simulink model "code"  (R2021b)
settings: Solver=FixedStepAuto  StartTime=0.0  StopTime=inf  RelTol=1e-3  EnableMultiTasking=on
libraries: vexarmcortexlib x5, vexcommonlib x2
settings Model: PacingRate=0.110000  Creator=mukul  LastModifiedBy=mukul
settings DataIOCC: LimitDataPoints=on  SignalLoggingSaveFormat=ModelDataLogs  ReturnWorkspaceOutputs=off
settings OptimizationCC: ExpressionDepthLimit=2147483647  LifeSpan=Inf  MaxStackSize=64  EfficientTunableParamExpr=on
settings DebuggingCC: UnderspecifiedInitializationDetection=Classic  MergeDetectMultiDrivingBlocksExec=none  InheritedTsInSrcMsg=none  FcnCallInpInsideContextMsg=warning  UnconnectedInputMsg=none  UnconnectedOutputMsg=none  StateNameClashWarn=warning  SFUnexpectedBacktrackingDiag=warning  SFNoUnconditionalDefaultTransitionDiag=warning  SFExecutionAtInitializationDiag=none  SFMachineParentedDataDiag=warning  ArithmeticOperatorsInVariantConditions=warning
settings HardwareCC: ProdBitPerPointer=32  ProdBitPerSizeT=32  ProdBitPerPtrDiffT=32  ProdLargestAtomicInteger=Long  ProdLargestAtomicFloat=Double  ProdIntDivRoundTo=Undefined  ProdWordSize=32  ProdHWDeviceType=ARM Compatible->ARM Cortex
settings ModelReferenceCC: PropagateSignalLabelsOutOfModel=off
settings SFSimCC: MATLABDynamicMemAlloc=off  CustomCodeUndefinedFunction=UseInterfaceOnly
settings RTWCC: Description=Embedded Coder  SystemTargetFile=ert.tlc  HardwareBoard=ARM Cortex-based VEX Microcontroller  TemplateMakefile=ert_default_tmf  Toolchain=GNU Tools for VEX ARM Cortex
settings CodeAppCC: IgnoreCustomStorageClasses=off  CustomSymbolStrType=$N$R$M  StateflowObjectComments=on  InternalIdentifier=Classic
settings ERTTargetCC: CodeReplacementLibrary=GCC ARM Cortex-M3  MultiwordLength=2048  ConvertIfToSwitch=off  SuppressUnreachableDefaultCases=off

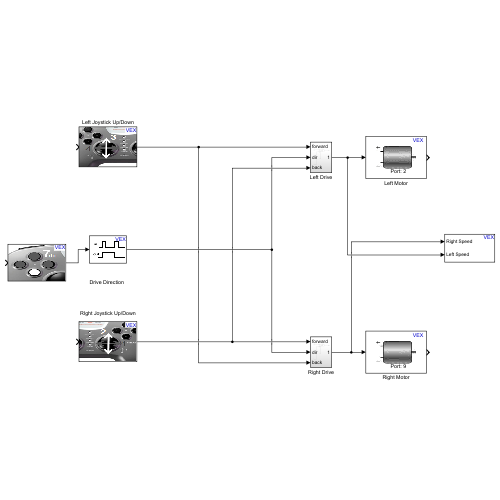
[thumbnail: Simulink's stored preview of the top-level diagram]
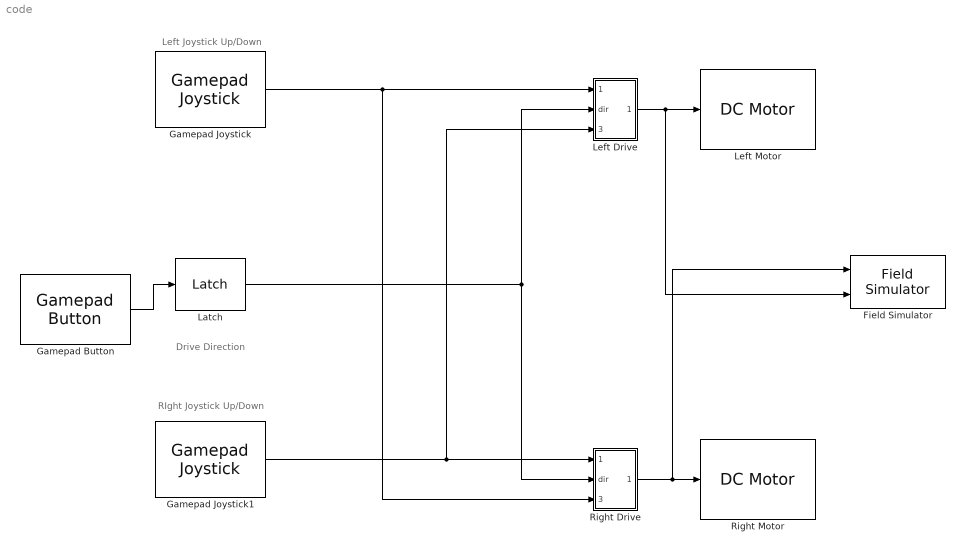
== system code ==
  note: RIght Joystick Up/Down
  note: Left Joystick Up/Down
  note: Drive Direction
  Field Simulator : vexcommonlib/Field Simulator  radius=2.5  space=10  range=200  BlockPlatform=vexarmcortex
      settings: SourceProductBaseCode=EC_VEX_MICRO,VEXV5
  Gamepad Button : vexarmcortexlib/Gamepad/Gamepad Button  joystick=1  chan=7  button56=Up  button78=Down  SimulationIn=on  SampleTime=0.02
      settings: SourceProductBaseCode=EC_VEX_MICRO
  Gamepad Joystick : vexarmcortexlib/Gamepad/Gamepad Joystick  joystick=1  chan=3  SimulationIn=on  SampleTime=0.02
      settings: SourceProductBaseCode=EC_VEX_MICRO
  Gamepad Joystick1 : vexarmcortexlib/Gamepad/Gamepad Joystick  joystick=1  chan=2  SimulationIn=on  SampleTime=0.02
      settings: SourceProductBaseCode=EC_VEX_MICRO
  Latch : vexcommonlib/Latch  output0=on  BlockPlatform=vexarmcortex
      settings: SourceProductBaseCode=EC_VEX_MICRO,VEXV5
  Left Drive : Subsystem
  Left Motor : vexarmcortexlib/Actuators/DC Motor  motor=2  scaleFactor=1/13.5  SimulationOut=on
      settings: SourceProductBaseCode=EC_VEX_MICRO
  Right Drive : Subsystem
  Right Motor : vexarmcortexlib/Actuators/DC Motor  motor=9  scaleFactor=1/13.5  SimulationOut=on
      settings: SourceProductBaseCode=EC_VEX_MICRO
  wires:
  Gamepad Button/1 -> Latch/1
  Gamepad Joystick1/1 -> Right Drive/1(forward), Left Drive/3(back)
  Gamepad Joystick/1 -> Right Drive/3(back), Left Drive/1(forward)
  Right Drive/1(Out1) -> Field Simulator/1, Right Motor/1
  Latch/1 -> Left Drive/2(dir), Right Drive/2(dir)
  Left Drive/1(Out1) -> Field Simulator/2, Left Motor/1

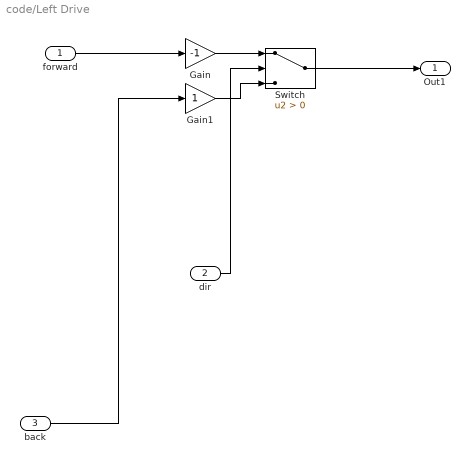
== system code/Left Drive ==
  forward : Inport
  dir : Inport  Port=2
  back : Inport  Port=3
  Gain : Gain  Gain=-1
  Gain1 : Gain
  Switch : Switch  Criteria=u2 > Threshold
  Out1 : Outport
  wires:
  back/1 -> Gain1/1
  Gain/1 -> Switch/1
  Gain1/1 -> Switch/3
  Switch/1 -> Out1/1
  forward/1 -> Gain/1
  dir/1 -> Switch/2

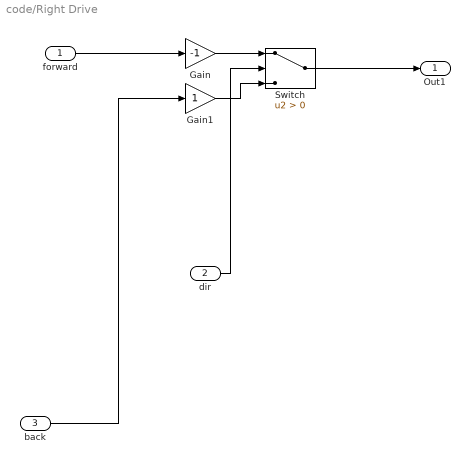
== system code/Right Drive ==
  forward : Inport
  dir : Inport  Port=2
  back : Inport  Port=3
  Gain : Gain  Gain=-1
  Gain1 : Gain
  Switch : Switch  Criteria=u2 > Threshold
  Out1 : Outport
  wires:
  back/1 -> Gain1/1
  Gain/1 -> Switch/1
  Gain1/1 -> Switch/3
  Switch/1 -> Out1/1
  forward/1 -> Gain/1
  dir/1 -> Switch/2
